simulink model "FlightControlSoftware"  (R2024a)
settings: Solver=VariableStepAuto  StartTime=0.0  StopTime=50  RelTol=1e-3
PreLoadFcn:
  | load Data/PropData.mat;
undefined symbols (not defined in the file): PropData
libraries: slpidlib x1
settings Model: Creator=callie  LastModifiedBy=callie

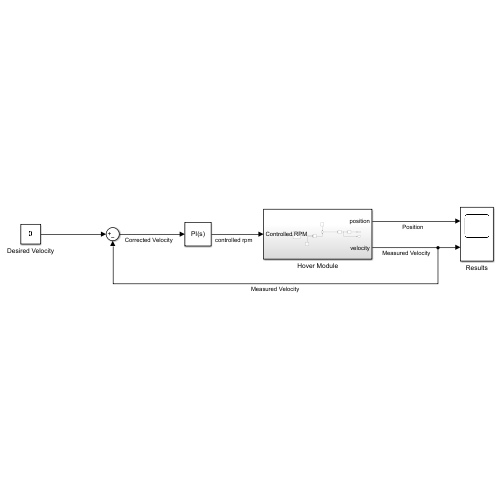
[thumbnail: Simulink's stored preview of the top-level diagram]
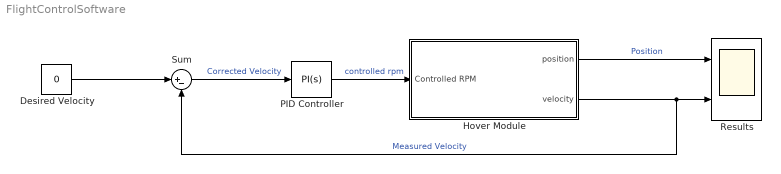
== system FlightControlSoftware ==
  Desired Velocity : Constant  Value=0
  Hover Module : Subsystem
  PID Controller : slpidlib/PID Controller  Controller=PI  Form=Parallel  TimeDomain=Continuous-time  UseExternalTs=off  SampleTime=-1  IntegratorMethod=Forward Euler  FilterMethod=Forward Euler  ControllerParametersSource=internal  P=28063.2903681465  I=4699.00310117393  UseKiTs=off  D=0  UseExternalDerivativeSource=off  N=100  UseFilter=on  TunerSelectOption=Transfer Function Based (PID Tuner App)  InitialConditionSource=internal  InitialConditionForIntegrator=0  InitialConditionForFilter=0  DifferentiatorICPrevScaledInput=0  ExternalReset=none  TrackingMode=off  Kt=1  LimitOutput=off  SatLimitsSource=internal  UpperSaturationLimit=inf  LowerSaturationLimit=-inf  LinearizeAsGain=on  AntiWindupMode=none  Kb=1  LimitIntegrator=off  UpperIntegratorSaturationLimit=inf  LowerIntegratorSaturationLimit=-inf  POutMin=[]  POutMax=[]  IOutMin=[]  IOutMax=[]  DOutMin=[]  DOutMax=[]  NOutMin=[]  NOutMax=[]  SumOutMin=[]  SumOutMax=[]  SaturationOutMin=[]  SaturationOutMax=[]  PParamMin=[]  PParamMax=[]  IParamMin=[]  IParamMax=[]  DParamMin=[]  DParamMax=[]  NParamMin=[]  NParamMax=[]  KbParamMin=[]  KbParamMax=[]  KtParamMin=[]  KtParamMax=[]  KbOutMin=[]  KbOutMax=[]  KtOutMin=[]  KtOutMax=[]  IntegratorOutMin=[]  IntegratorOutMax=[]  FilterOutMin=[]  FilterOutMax=[]  SumI1OutMin=[]  SumI1OutMax=[]  SumI2OutMin=[]  SumI2OutMax=[]  SumI3OutMin=[]  SumI3OutMax=[]  SumI4OutMin=[]  SumI4OutMax=[]  SumDOutMin=[]  SumDOutMax=[]  DifferentiatorOutMin=[]  DifferentiatorOutMax=[]  FilterDiffOutCoefMin=[]  FilterDiffOutCoefMax=[]  ReciprocalOutMin=[]  ReciprocalOutMax=[]  SumDenOutMin=[]  SumDenOutMax=[]  SumNumOutMin=[]  SumNumOutMax=[]  DivideOutMin=[]  DivideOutMax=[]  UdiffTsProdOutMin=[]  UdiffTsProdOutMax=[]  NTsProdOutMin=[]  NTsProdOutMax=[]  UintegralTsProdOutMin=[]  UintegralTsProdOutMax=[]  UngainTsProdOutMin=[]  UngainTsProdOutMax=[]  ClampingZeroOutDataTypeStr=Inherit: Inherit via back propagation  ClampingZeroOutMin=[]  ClampingZeroOutMax=[]  FilterDenConstantOutDataTypeStr=Inherit: Inherit via back propagation  FilterDenConstantOutMin=[]  FilterDenConstantOutMax=[]  PCopyOutDataTypeStr=Inherit: Inherit via back propagation  PCopyOutMin=[]  PCopyOutMax=[]  NCopyOutDataTypeStr=Inherit: Inherit via back propagation  NCopyOutMin=[]  NCopyOutMax=[]  IntegratorContinuousStateAttributes=''  IntegratorStateMustResolveToSignalObject=off  IntegratorRTWStateStorageClass=Auto  FilterContinuousStateAttributes=''  FilterStateMustResolveToSignalObject=off  FilterRTWStateStorageClass=Auto  ParallelPVariant=InternalParameters  IdealPVariant=Disabled  IVariant=InternalParameters  DVariant=Disabled  IntegratorVariant=Continuous  SatVariant=Disabled  AWVariant=Passthrough  PCopyVariant=Disabled  TRVariant=Disabled  FdbkBlocksVariant=Forward  IdealPFdbkVariant=Disabled  SatFdbkVariant=Disabled  DerivativeFilterVariant=Disabled  NVariant=Disabled  NCopyVariant=Disabled_SignalSpec  FilterICVariant=Disabled  IntegratorICVariant=InternalICs  ExternalResetVariant=Disabled  TRSumVariant=Passthrough  SumFdbkVariant=Disabled  SumVariant=Sum_PI  TsampFilterVariant=InternalTs  TsampNgainVariant=Passthrough  TsampIntegralVariant=Disabled_SignalSpec  ExternalSaturationOutDataTypeStr=Inherit: Same as second input  DerivativeSourceVariant=Disabled
  Results : Scope  NumInputPorts=2
  Sum : Sum  Inputs=|+-
  wires:
  PID Controller/1 -> Hover Module/1(Controlled RPM)  "controlled rpm"
  Hover Module/1(position) -> Results/1  "Position"
  Sum/1 -> PID Controller/1  "Corrected Velocity"
  Hover Module/2(velocity) -> Sum/2, Results/2  "Measured Velocity"
  Desired Velocity/1 -> Sum/1

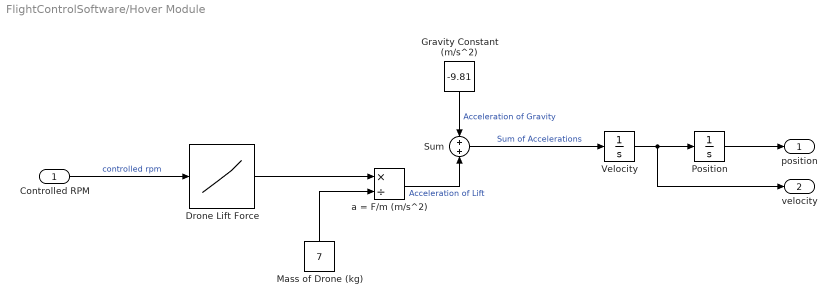
== system FlightControlSoftware/Hover Module ==
  Controlled RPM : Inport
  Drone Lift Force : Lookup_n-D  NumberOfTableDimensions=1  BreakpointsForDimension1=PropData.rpm  Table=PropData.lift  InternalRulePriority=Speed  RndMeth=Simplest
  Gravity Constant (m/s^2) : Constant  Value=-9.81
  Mass of Drone (kg) : Constant  Value=7
  Position : Integrator  InitialCondition=15
  Sum : Sum  Inputs=+|+
  Velocity : Integrator
  a = F/m (m/s^2) : Product  Inputs=*/
  position : Outport  VectorParamsAs1DForOutWhenUnconnected=off
  velocity : Outport  Port=2  VectorParamsAs1DForOutWhenUnconnected=off
  wires:
  Controlled RPM/1 -> Drone Lift Force/1  "controlled rpm"
  Drone Lift Force/1 -> a = F/m (m/s^2)/1
  Velocity/1 -> Position/1, velocity/1
  Sum/1 -> Velocity/1  "Sum of Accelerations"
  Position/1 -> position/1
  a = F/m (m/s^2)/1 -> Sum/2  "Acceleration of Lift"
  Gravity Constant (m/s^2)/1 -> Sum/1  "Acceleration of Gravity"
  Mass of Drone (kg)/1 -> a = F/m (m/s^2)/2
